simulink model "confirmacao_linearizacao"  (R2018a)
settings: Solver=FixedStepAuto  StartTime=0.0  StopTime=tfinal  FixedStep=dt  RelTol=1e-3
values from neighbouring files (symbols this model uses):
  a1 = 0.0190125110732    [PSO_workspace_PID_v1.0_agoravai_refnova.mat]    (also in cobem_IMC_script.m; teste_linearizacao.m)
  a2 = 0.594107643424    [PSO_workspace_PID_v1.0_agoravai_refnova.mat]    (also in cobem_IMC_script.m = num2/den2; teste_linearizacao.m = num2/den2)
  a3 = 0.0893725569407    [PSO_workspace_PID_v1.0_agoravai_refnova.mat]    (also in cobem_IMC_script.m = num3/den3; teste_linearizacao.m = num3/den3)
  a4 = 0.0670294177055    [PSO_workspace_PID_v1.0_agoravai_refnova.mat]    (also in cobem_IMC_script.m = num4/den4; teste_linearizacao.m = num4/den4)
  H1max = 1    [PSO_workspace_PID_v1.0_agoravai_refnova.mat]    (also in cobem_IMC_script.m; teste_linearizacao.m)
  H2max = 1    [PSO_workspace_PID_v1.0_agoravai_refnova.mat]    (also in cobem_IMC_script.m; teste_linearizacao.m)
undefined symbols (not defined in the file or in its folder): den, num
settings Model: Creator=generic-user  LastModifiedBy=generic-user

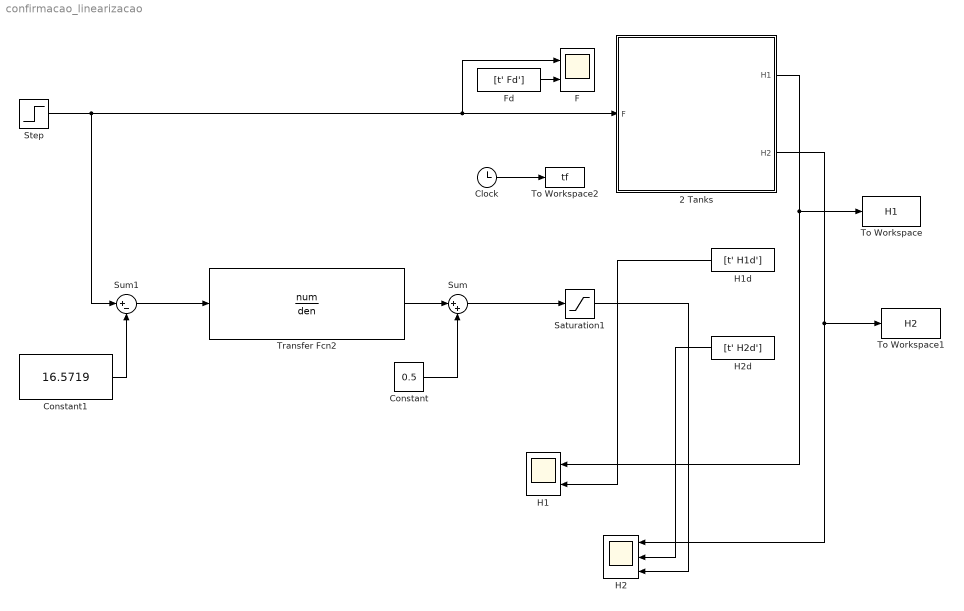
== system confirmacao_linearizacao ==
  2 Tanks : Subsystem
  Clock : Clock
  Constant : Constant  Value=0.5
  Constant1 : Constant  Value=16.5719
  F : Scope  NumInputPorts=2
  Fd : FromWorkspace  VariableName=[t' Fd']  SampleTime=0  OutputAfterFinalValue=Holding final value
  H1 : Scope  NumInputPorts=2
  H1d : FromWorkspace  VariableName=[t' H1d']  SampleTime=0  OutputAfterFinalValue=Holding final value
  H2 : Scope  NumInputPorts=3
  H2d : FromWorkspace  VariableName=[t' H2d']  SampleTime=0  OutputAfterFinalValue=Holding final value
  Saturation1 : Saturate  UpperLimit=H2max  LowerLimit=0
  Step : Step  Time=0  After=16.75  SampleTime=0
  Sum : Sum  Inputs=|++
  Sum1 : Sum  Inputs=|+-
  To Workspace : ToWorkspace  VariableName=H1  SampleTime=-1
  To Workspace1 : ToWorkspace  VariableName=H2  SampleTime=-1
  To Workspace2 : ToWorkspace  VariableName=tf  SampleTime=-1
  Transfer Fcn2 : TransferFcn  Numerator=num  Denominator=den
  wires:
  Step/1 -> Sum1/1, F/1, 2 Tanks/1(F)
  2 Tanks/1(H1) -> To Workspace/1, H1/1
  H2d/1 -> H2/2
  H1d/1 -> H1/2
  2 Tanks/2(H2) -> To Workspace1/1, H2/1
  Clock/1 -> To Workspace2/1
  Fd/1 -> F/2
  Saturation1/1 -> H2/3
  Transfer Fcn2/1 -> Sum/1
  Sum/1 -> Saturation1/1
  Constant/1 -> Sum/2
  Sum1/1 -> Transfer Fcn2/1
  Constant1/1 -> Sum1/2

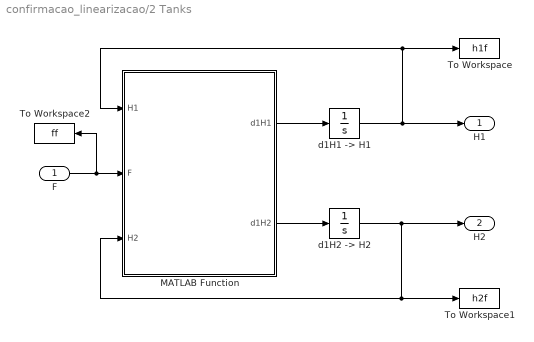
== system confirmacao_linearizacao/2 Tanks ==
  F : Inport
  MATLAB Function : MATLAB Function  TreatAsAtomicUnit=on
  To Workspace : ToWorkspace  VariableName=h1f  SampleTime=-1
  To Workspace1 : ToWorkspace  VariableName=h2f  SampleTime=-1
  To Workspace2 : ToWorkspace  VariableName=ff  SampleTime=-1
  "d1H1 -> H1" : Integrator  InitialCondition=0.2813  LimitOutput=on  UpperSaturationLimit=H1max  LowerSaturationLimit=0
  "d1H2 -> H2" : Integrator  InitialCondition=0.5  LimitOutput=on  UpperSaturationLimit=H2max  LowerSaturationLimit=0
  H1 : Outport
  H2 : Outport  Port=2
  wires:
  MATLAB Function/1(d1H1) -> "d1H1 -> H1"/1
  "d1H1 -> H1"/1 -> H1/1, To Workspace/1, MATLAB Function/1(H1)
  MATLAB Function/2(d1H2) -> "d1H2 -> H2"/1
  F/1 -> To Workspace2/1, MATLAB Function/2(F)
  "d1H2 -> H2"/1 -> H2/1, To Workspace1/1, MATLAB Function/3(H2)

== matlab function confirmacao_linearizacao/2 Tanks/MATLAB Function ==
  data: H1 input; F input; d1H1 output; H2 input; d1H2 output; a1 parameter; a2 parameter; a3 parameter; a4 parameter
function [d1H1, d1H2] = TwoTanks(H1, F, H2, a1, a2, a3, a4)
  
  % Sistema Dinâmico
    d1H1 = a1*F - a2*sqrt(H1);
    
    d1H2 = a3*(sqrt(H1)/(H2^2)) - a4*(1/(H2^1.5));
